simulink model "poco_ref_al_r307"  (Simulink 6.2)
settings: Solver=ode45  StartTime=0.0  StopTime=100000  RelTol=1e-3
libraries: xbsIndex_r3 x1012, xps_library x42, ddc_library x4, adcscope_lib x2, fft_library x2, pfb_library x2, delay_lib x1
(part 7 of 9)

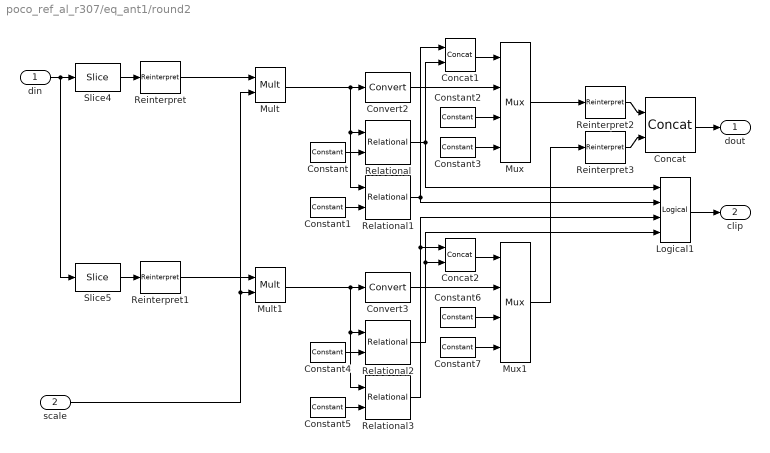
== system poco_ref_al_r307/eq_ant1/round2 ==
  din : Inport  Port=1  LatchInput=off
  scale : Inport  Port=2  LatchInput=off
  Concat : xbsIndex_r3/Concat  num_inputs=2  explicit_period=off  period=1  dbl_ovrd=off
  Concat1 : xbsIndex_r3/Concat  num_inputs=2  explicit_period=off  period=1  dbl_ovrd=off
  Concat2 : xbsIndex_r3/Concat  num_inputs=2  explicit_period=off  period=1  dbl_ovrd=off
  Constant : xbsIndex_r3/Constant  const=7/8  equ=P=C  arith_type="Signed  (2's comp)"  n_bits=27  bin_pt=18  opselect=C  inp2=PCIN>>17  opr=+  inp1=P  carry=CIN  iostate=0  explicit_period=on  period=1  dbl_ovrd=off
  Constant1 : xbsIndex_r3/Constant  const=-7/8  equ=P=C  arith_type="Signed  (2's comp)"  n_bits=27  bin_pt=18  opselect=C  inp2=PCIN>>17  opr=+  inp1=P  carry=CIN  iostate=0  explicit_period=on  period=1  dbl_ovrd=off
  Constant2 : xbsIndex_r3/Constant  const=7/8  equ=P=C  arith_type="Signed  (2's comp)"  n_bits=4  bin_pt=3  opselect=C  inp2=PCIN>>17  opr=+  inp1=P  carry=CIN  iostate=0  explicit_period=on  period=1  dbl_ovrd=off
  Constant3 : xbsIndex_r3/Constant  const=-7/8  equ=P=C  arith_type="Signed  (2's comp)"  n_bits=4  bin_pt=3  opselect=C  inp2=PCIN>>17  opr=+  inp1=P  carry=CIN  iostate=0  explicit_period=on  period=1  dbl_ovrd=off
  Constant4 : xbsIndex_r3/Constant  const=7/8  equ=P=C  arith_type="Signed  (2's comp)"  n_bits=27  bin_pt=18  opselect=C  inp2=PCIN>>17  opr=+  inp1=P  carry=CIN  iostate=0  explicit_period=on  period=1  dbl_ovrd=off
  Constant5 : xbsIndex_r3/Constant  const=-7/8  equ=P=C  arith_type="Signed  (2's comp)"  n_bits=27  bin_pt=18  opselect=C  inp2=PCIN>>17  opr=+  inp1=P  carry=CIN  iostate=0  explicit_period=on  period=1  dbl_ovrd=off
  Constant6 : xbsIndex_r3/Constant  const=7/8  equ=P=C  arith_type="Signed  (2's comp)"  n_bits=4  bin_pt=3  opselect=C  inp2=PCIN>>17  opr=+  inp1=P  carry=CIN  iostate=0  explicit_period=on  period=1  dbl_ovrd=off
  Constant7 : xbsIndex_r3/Constant  const=-7/8  equ=P=C  arith_type="Signed  (2's comp)"  n_bits=4  bin_pt=3  opselect=C  inp2=PCIN>>17  opr=+  inp1=P  carry=CIN  iostate=0  explicit_period=on  period=1  dbl_ovrd=off
  Convert2 : xbsIndex_r3/Convert  arith_type="Signed  (2's comp)"  n_bits=4  bin_pt=3  quantization="Round  (unbiased: Even Values)"  overflow=Wrap  latency=2  explicit_period=off  period=1  dbl_ovrd=off  show_param=off  inserted_by_tool=off  pipeline=off
      settings: xl_area=[0, 0, 0, 0, 0, 0, 0]
  Convert3 : xbsIndex_r3/Convert  arith_type="Signed  (2's comp)"  n_bits=4  bin_pt=3  quantization="Round  (unbiased: Even Values)"  overflow=Wrap  latency=2  explicit_period=off  period=1  dbl_ovrd=off  show_param=off  inserted_by_tool=off  pipeline=off
      settings: xl_area=[0, 0, 0, 0, 0, 0, 0]
  Logical1 : xbsIndex_r3/Logical  logical_function=OR  inputs=4  precision=Full  arith_type=Unsigned  n_bits=8  bin_pt=2  align_bp=on  latency=2  explicit_period=off  period=1  en=off  dbl_ovrd=off  show_param=off
      settings: xl_area=[0, 0, 0, 0, 0, 0, 0]
  Mult : xbsIndex_r3/Mult  precision=Full  arith_type="Signed  (2's comp)"  n_bits=8  bin_pt=2  quantization=Truncate  overflow=Wrap  latency=2  explicit_period=off  period=1  en=off  dbl_ovrd=off  show_param=on  mult_type=Parallel  oversample=2  use_embedded=on  pipeline=on  use_rpm=on  placement_style=Rectangular Shape  gen_core=off
      settings: xl_area=[0, 0, 0, 0, 0, 0, 0]
  Mult1 : xbsIndex_r3/Mult  precision=Full  arith_type="Signed  (2's comp)"  n_bits=8  bin_pt=2  quantization=Truncate  overflow=Wrap  latency=2  explicit_period=off  period=1  en=off  dbl_ovrd=off  show_param=on  mult_type=Parallel  oversample=2  use_embedded=on  pipeline=on  use_rpm=on  placement_style=Rectangular Shape  gen_core=off
      settings: xl_area=[0, 0, 0, 0, 0, 0, 0]
  Mux : xbsIndex_r3/Mux  inputs=3  precision=Full  arith_type="Signed  (2's comp)"  n_bits=8  bin_pt=2  quantization=Truncate  overflow=Wrap  latency=0  explicit_period=off  period=1  en=off  dbl_ovrd=off  show_param=off  mux_type=off  use_rpm=off  gen_core=off
      settings: xl_area=[0, 0, 0, 0, 0, 0, 0]
  Mux1 : xbsIndex_r3/Mux  inputs=3  precision=Full  arith_type="Signed  (2's comp)"  n_bits=8  bin_pt=2  quantization=Truncate  overflow=Wrap  latency=0  explicit_period=off  period=1  en=off  dbl_ovrd=off  show_param=off  mux_type=off  use_rpm=off  gen_core=off
      settings: xl_area=[0, 0, 0, 0, 0, 0, 0]
  Reinterpret : xbsIndex_r3/Reinterpret  force_arith_type=on  arith_type="Signed  (2's comp)"  force_bin_pt=on  bin_pt=17  force_valid=on
  Reinterpret1 : xbsIndex_r3/Reinterpret  force_arith_type=on  arith_type="Signed  (2's comp)"  force_bin_pt=on  bin_pt=17  force_valid=on
  Reinterpret2 : xbsIndex_r3/Reinterpret  force_arith_type=on  arith_type=Unsigned  force_bin_pt=on  bin_pt=0  force_valid=on
  Reinterpret3 : xbsIndex_r3/Reinterpret  force_arith_type=on  arith_type=Unsigned  force_bin_pt=on  bin_pt=0  force_valid=on
  Relational : xbsIndex_r3/Relational  mode=a>b  latency=2  explicit_period=off  period=1  en=off  dbl_ovrd=off  show_param=off
      settings: xl_area=[0, 0, 0, 0, 0, 0, 0]
  Relational1 : xbsIndex_r3/Relational  mode=a<b  latency=2  explicit_period=off  period=1  en=off  dbl_ovrd=off  show_param=off
      settings: xl_area=[0, 0, 0, 0, 0, 0, 0]
  Relational2 : xbsIndex_r3/Relational  mode=a>b  latency=2  explicit_period=off  period=1  en=off  dbl_ovrd=off  show_param=off
      settings: xl_area=[0, 0, 0, 0, 0, 0, 0]
  Relational3 : xbsIndex_r3/Relational  mode=a<b  latency=2  explicit_period=off  period=1  en=off  dbl_ovrd=off  show_param=off
      settings: xl_area=[0, 0, 0, 0, 0, 0, 0]
  Slice4 : xbsIndex_r3/Slice  mode=Upper Bit Location + Width  nbits=18  bit1=0  base1=MSB of Input  bit0=0  base0=LSB of Input  boolean_output=off  explicit_period=off  period=1  dbl_ovrd=off
  Slice5 : xbsIndex_r3/Slice  mode=Lower Bit Location + Width  nbits=18  bit1=0  base1=MSB of Input  bit0=0  base0=LSB of Input  boolean_output=off  explicit_period=off  period=1  dbl_ovrd=off
  dout : Outport
  clip : Outport  Port=2
  wires:
  Logical1/1 -> clip/1
  Mult/1 -> Relational1/1, Relational/1, Convert2/1
  Mult1/1 -> Relational3/1, Relational2/1, Convert3/1
  Mux1/1 -> Reinterpret3/1
  Mux/1 -> Reinterpret2/1
  Relational3/1 -> Logical1/3, Concat2/1
  Relational2/1 -> Logical1/4, Concat2/2
  Constant7/1 -> Mux1/4
  Constant6/1 -> Mux1/3
  Constant5/1 -> Relational3/2
  Constant4/1 -> Relational2/2
  Concat2/1 -> Mux1/1
  Convert3/1 -> Mux1/2
  Relational1/1 -> Logical1/2, Concat1/1
  Relational/1 -> Logical1/1, Concat1/2
  Constant3/1 -> Mux/4
  Constant2/1 -> Mux/3
  Constant1/1 -> Relational1/2
  Constant/1 -> Relational/2
  Concat1/1 -> Mux/1
  Convert2/1 -> Mux/2
  scale/1 -> Mult/2, Mult1/2
  Reinterpret/1 -> Mult/1
  Reinterpret1/1 -> Mult1/1
  Concat/1 -> dout/1
  din/1 -> Slice5/1, Slice4/1
  Reinterpret3/1 -> Concat/2
  Slice5/1 -> Reinterpret1/1
  Reinterpret2/1 -> Concat/1
  Slice4/1 -> Reinterpret/1

== system poco_ref_al_r307/pulse_ext1/posedge ==
  In : Inport  Port=1  LatchInput=off
  Delay : xbsIndex_r3/Delay  latency=1  reg_retiming=off  explicit_period=off  period=1  en=off  accept_only_valid=off  init_zero=on  dbl_ovrd=off  show_param=off
      settings: xl_area=[0, 0, 0, 0, 0, 0, 0]
  Inverter : xbsIndex_r3/Inverter  latency=0  explicit_period=off  period=1  en=off  dbl_ovrd=off  show_param=off
      settings: xl_area=[0, 0, 0, 0, 0, 0, 0]
  Logical : xbsIndex_r3/Logical  logical_function=AND  inputs=2  precision=Full  arith_type=Unsigned  n_bits=8  bin_pt=2  align_bp=on  latency=0  explicit_period=off  period=1  en=off  dbl_ovrd=off  show_param=off
      settings: xl_area=[0, 0, 0, 0, 0, 0, 0]
  Out : Outport
  wires:
  Logical/1 -> Out/1
  In/1 -> Logical/2, Delay/1
  Inverter/1 -> Logical/1
  Delay/1 -> Inverter/1

== system poco_ref_al_r307/pulse_ext2/posedge ==
  In : Inport  Port=1  LatchInput=off
  Delay : xbsIndex_r3/Delay  latency=1  reg_retiming=off  explicit_period=off  period=1  en=off  accept_only_valid=off  init_zero=on  dbl_ovrd=off  show_param=off
      settings: xl_area=[0, 0, 0, 0, 0, 0, 0]
  Inverter : xbsIndex_r3/Inverter  latency=0  explicit_period=off  period=1  en=off  dbl_ovrd=off  show_param=off
      settings: xl_area=[0, 0, 0, 0, 0, 0, 0]
  Logical : xbsIndex_r3/Logical  logical_function=AND  inputs=2  precision=Full  arith_type=Unsigned  n_bits=8  bin_pt=2  align_bp=on  latency=0  explicit_period=off  period=1  en=off  dbl_ovrd=off  show_param=off
      settings: xl_area=[0, 0, 0, 0, 0, 0, 0]
  Out : Outport
  wires:
  Delay/1 -> Inverter/1
  Inverter/1 -> Logical/1
  In/1 -> Delay/1, Logical/2
  Logical/1 -> Out/1

== system poco_ref_al_r307/pulse_ext3/posedge ==
  In : Inport  Port=1  LatchInput=off
  Delay : xbsIndex_r3/Delay  latency=1  reg_retiming=off  explicit_period=off  period=1  en=off  accept_only_valid=off  init_zero=on  dbl_ovrd=off  show_param=off
      settings: xl_area=[0, 0, 0, 0, 0, 0, 0]
  Inverter : xbsIndex_r3/Inverter  latency=0  explicit_period=off  period=1  en=off  dbl_ovrd=off  show_param=off
      settings: xl_area=[0, 0, 0, 0, 0, 0, 0]
  Logical : xbsIndex_r3/Logical  logical_function=AND  inputs=2  precision=Full  arith_type=Unsigned  n_bits=8  bin_pt=2  align_bp=on  latency=0  explicit_period=off  period=1  en=off  dbl_ovrd=off  show_param=off
      settings: xl_area=[0, 0, 0, 0, 0, 0, 0]
  Out : Outport
  wires:
  Delay/1 -> Inverter/1
  Inverter/1 -> Logical/1
  In/1 -> Delay/1, Logical/2
  Logical/1 -> Out/1

== system poco_ref_al_r307/pulse_ext4/posedge ==
  In : Inport  Port=1  LatchInput=off
  Delay : xbsIndex_r3/Delay  latency=1  reg_retiming=off  explicit_period=off  period=1  en=off  accept_only_valid=off  init_zero=on  dbl_ovrd=off  show_param=off
      settings: xl_area=[0, 0, 0, 0, 0, 0, 0]
  Inverter : xbsIndex_r3/Inverter  latency=0  explicit_period=off  period=1  en=off  dbl_ovrd=off  show_param=off
      settings: xl_area=[0, 0, 0, 0, 0, 0, 0]
  Logical : xbsIndex_r3/Logical  logical_function=AND  inputs=2  precision=Full  arith_type=Unsigned  n_bits=8  bin_pt=2  align_bp=on  latency=0  explicit_period=off  period=1  en=off  dbl_ovrd=off  show_param=off
      settings: xl_area=[0, 0, 0, 0, 0, 0, 0]
  Out : Outport
  wires:
  Delay/1 -> Inverter/1
  Inverter/1 -> Logical/1
  In/1 -> Delay/1, Logical/2
  Logical/1 -> Out/1

== system poco_ref_al_r307/pulse_ext5/posedge ==
  In : Inport  Port=1  LatchInput=off
  Delay : xbsIndex_r3/Delay  latency=1  reg_retiming=off  explicit_period=off  period=1  en=off  accept_only_valid=off  init_zero=on  dbl_ovrd=off  show_param=off
      settings: xl_area=[0, 0, 0, 0, 0, 0, 0]
  Inverter : xbsIndex_r3/Inverter  latency=0  explicit_period=off  period=1  en=off  dbl_ovrd=off  show_param=off
      settings: xl_area=[0, 0, 0, 0, 0, 0, 0]
  Logical : xbsIndex_r3/Logical  logical_function=AND  inputs=2  precision=Full  arith_type=Unsigned  n_bits=8  bin_pt=2  align_bp=on  latency=0  explicit_period=off  period=1  en=off  dbl_ovrd=off  show_param=off
      settings: xl_area=[0, 0, 0, 0, 0, 0, 0]
  Out : Outport
  wires:
  Logical/1 -> Out/1
  In/1 -> Logical/2, Delay/1
  Inverter/1 -> Logical/1
  Delay/1 -> Inverter/1

== system poco_ref_al_r307/pulse_ext6/posedge ==
  In : Inport  Port=1  LatchInput=off
  Delay : xbsIndex_r3/Delay  latency=1  reg_retiming=off  explicit_period=off  period=1  en=off  accept_only_valid=off  init_zero=on  dbl_ovrd=off  show_param=off
      settings: xl_area=[0, 0, 0, 0, 0, 0, 0]
  Inverter : xbsIndex_r3/Inverter  latency=0  explicit_period=off  period=1  en=off  dbl_ovrd=off  show_param=off
      settings: xl_area=[0, 0, 0, 0, 0, 0, 0]
  Logical : xbsIndex_r3/Logical  logical_function=AND  inputs=2  precision=Full  arith_type=Unsigned  n_bits=8  bin_pt=2  align_bp=on  latency=0  explicit_period=off  period=1  en=off  dbl_ovrd=off  show_param=off
      settings: xl_area=[0, 0, 0, 0, 0, 0, 0]
  Out : Outport
  wires:
  Logical/1 -> Out/1
  In/1 -> Logical/2, Delay/1
  Inverter/1 -> Logical/1
  Delay/1 -> Inverter/1

== system poco_ref_al_r307/pulse_ext7/posedge ==
  In : Inport  Port=1  LatchInput=off
  Delay : xbsIndex_r3/Delay  latency=1  reg_retiming=off  explicit_period=off  period=1  en=off  accept_only_valid=off  init_zero=on  dbl_ovrd=off  show_param=off
      settings: xl_area=[0, 0, 0, 0, 0, 0, 0]
  Inverter : xbsIndex_r3/Inverter  latency=0  explicit_period=off  period=1  en=off  dbl_ovrd=off  show_param=off
      settings: xl_area=[0, 0, 0, 0, 0, 0, 0]
  Logical : xbsIndex_r3/Logical  logical_function=AND  inputs=2  precision=Full  arith_type=Unsigned  n_bits=8  bin_pt=2  align_bp=on  latency=0  explicit_period=off  period=1  en=off  dbl_ovrd=off  show_param=off
      settings: xl_area=[0, 0, 0, 0, 0, 0, 0]
  Out : Outport
  wires:
  Logical/1 -> Out/1
  In/1 -> Logical/2, Delay/1
  Inverter/1 -> Logical/1
  Delay/1 -> Inverter/1

== system poco_ref_al_r307/sync_gen/edge ==
  in : Inport  Port=1  LatchInput=off
  Delay4 : xbsIndex_r3/Delay  latency=1  reg_retiming=off  explicit_period=off  period=1  en=off  accept_only_valid=off  init_zero=on  dbl_ovrd=off  show_param=off
      settings: xl_area=[0, 0, 0, 0, 0, 0, 0]
  Logical3 : xbsIndex_r3/Logical  logical_function=XOR  inputs=2  precision=Full  arith_type=Unsigned  n_bits=8  bin_pt=2  align_bp=on  latency=0  explicit_period=off  period=1  en=off  dbl_ovrd=off  show_param=off
      settings: xl_area=[0, 0, 0, 0, 0, 0, 0]
  out : Outport
  wires:
  Logical3/1 -> out/1
  Delay4/1 -> Logical3/1
  in/1 -> Delay4/1, Logical3/2

== system poco_ref_al_r307/sync_gen/posedge1 ==
  In : Inport  Port=1  LatchInput=off
  Delay : xbsIndex_r3/Delay  latency=1  reg_retiming=off  explicit_period=off  period=1  en=off  accept_only_valid=off  init_zero=on  dbl_ovrd=off  show_param=off
      settings: xl_area=[0, 0, 0, 0, 0, 0, 0]
  Inverter : xbsIndex_r3/Inverter  latency=0  explicit_period=off  period=1  en=off  dbl_ovrd=off  show_param=off
      settings: xl_area=[0, 0, 0, 0, 0, 0, 0]
  Logical : xbsIndex_r3/Logical  logical_function=AND  inputs=2  precision=Full  arith_type=Unsigned  n_bits=8  bin_pt=2  align_bp=on  latency=0  explicit_period=off  period=1  en=off  dbl_ovrd=off  show_param=off
      settings: xl_area=[0, 0, 0, 0, 0, 0, 0]
  Out : Outport
  wires:
  Logical/1 -> Out/1
  In/1 -> Logical/2, Delay/1
  Inverter/1 -> Logical/1
  Delay/1 -> Inverter/1

== system poco_ref_al_r307/sync_gen/posedge2 ==
  In : Inport  Port=1  LatchInput=off
  Delay : xbsIndex_r3/Delay  latency=1  reg_retiming=off  explicit_period=off  period=1  en=off  accept_only_valid=off  init_zero=on  dbl_ovrd=off  show_param=off
      settings: xl_area=[0, 0, 0, 0, 0, 0, 0]
  Inverter : xbsIndex_r3/Inverter  latency=0  explicit_period=off  period=1  en=off  dbl_ovrd=off  show_param=off
      settings: xl_area=[0, 0, 0, 0, 0, 0, 0]
  Logical : xbsIndex_r3/Logical  logical_function=AND  inputs=2  precision=Full  arith_type=Unsigned  n_bits=8  bin_pt=2  align_bp=on  latency=0  explicit_period=off  period=1  en=off  dbl_ovrd=off  show_param=off
      settings: xl_area=[0, 0, 0, 0, 0, 0, 0]
  Out : Outport
  wires:
  Delay/1 -> Inverter/1
  Inverter/1 -> Logical/1
  In/1 -> Delay/1, Logical/2
  Logical/1 -> Out/1

== system poco_ref_al_r307/dir_x/aa/c_to_ri ==
  c : Inport  Port=1  LatchInput=off
  force_im : xbsIndex_r3/Reinterpret  force_arith_type=on  arith_type="Signed  (2's comp)"  force_bin_pt=on  bin_pt=bin_pt  force_valid=on
  force_re : xbsIndex_r3/Reinterpret  force_arith_type=on  arith_type="Signed  (2's comp)"  force_bin_pt=on  bin_pt=bin_pt  force_valid=on
  slice_im : xbsIndex_r3/Slice  mode=Lower Bit Location + Width  nbits=n_bits  bit1=0  base1=MSB of Input  bit0=0  base0=LSB of Input  boolean_output=off  explicit_period=off  period=1  dbl_ovrd=off
  slice_re : xbsIndex_r3/Slice  mode=Upper Bit Location + Width  nbits=n_bits  bit1=0  base1=MSB of Input  bit0=0  base0=LSB of Input  boolean_output=off  explicit_period=off  period=1  dbl_ovrd=off
  re : Outport
  im : Outport  Port=2
  wires:
  slice_re/1 -> force_re/1
  slice_im/1 -> force_im/1
  force_re/1 -> re/1
  force_im/1 -> im/1
  c/1 -> slice_re/1, slice_im/1

== system poco_ref_al_r307/dir_x/aa/c_to_ri1 ==
  c : Inport  Port=1  LatchInput=off
  force_im : xbsIndex_r3/Reinterpret  force_arith_type=on  arith_type="Signed  (2's comp)"  force_bin_pt=on  bin_pt=bin_pt  force_valid=on
  force_re : xbsIndex_r3/Reinterpret  force_arith_type=on  arith_type="Signed  (2's comp)"  force_bin_pt=on  bin_pt=bin_pt  force_valid=on
  slice_im : xbsIndex_r3/Slice  mode=Lower Bit Location + Width  nbits=n_bits  bit1=0  base1=MSB of Input  bit0=0  base0=LSB of Input  boolean_output=off  explicit_period=off  period=1  dbl_ovrd=off
  slice_re : xbsIndex_r3/Slice  mode=Upper Bit Location + Width  nbits=n_bits  bit1=0  base1=MSB of Input  bit0=0  base0=LSB of Input  boolean_output=off  explicit_period=off  period=1  dbl_ovrd=off
  re : Outport
  im : Outport  Port=2
  wires:
  slice_re/1 -> force_re/1
  slice_im/1 -> force_im/1
  force_re/1 -> re/1
  force_im/1 -> im/1
  c/1 -> slice_re/1, slice_im/1

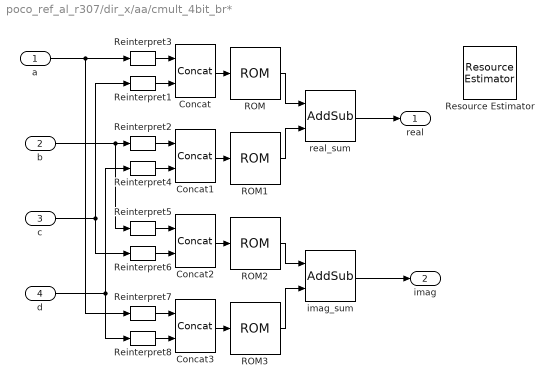
== system poco_ref_al_r307/dir_x/aa/cmult_4bit_br* ==
  a : Inport  Port=1  LatchInput=off
  b : Inport  Port=2  LatchInput=off
  c : Inport  Port=3  LatchInput=off
  d : Inport  Port=4  LatchInput=off
  Concat{,1..3} (4 alike) : xbsIndex_r3/Concat  num_inputs=2  explicit_period=off  period=1  dbl_ovrd=off
  ROM : xbsIndex_r3/ROM  depth=256  initVector=transpose(transpose([0:7 -8:-1]) * [0:7 -8:-1]) / 64  arith_type="Signed  (2's comp)"  n_bits=8  bin_pt=6  latency=mult_latency  init_zero=on  explicit_period=off  period=1  rst=off  init_reg=0  en=off  dbl_ovrd=off  show_param=off  distributed_mem=off  use_rpm=off  gen_core=off
      settings: xl_area=[0 0 1 0 0 0 0]
  ROM1 : xbsIndex_r3/ROM  depth=256  initVector=transpose([0:7 -8:-1]) * [0:7 -8:-1] / 64  arith_type="Signed  (2's comp)"  n_bits=8  bin_pt=6  latency=mult_latency  init_zero=on  explicit_period=off  period=1  rst=off  init_reg=0  en=off  dbl_ovrd=off  show_param=off  distributed_mem=off  use_rpm=off  gen_core=off
      settings: xl_area=[0 0 1 0 0 0 0]
  ROM2 : xbsIndex_r3/ROM  depth=256  initVector=transpose([0:7 -8:-1]) * [0:7 -8:-1] / 64  arith_type="Signed  (2's comp)"  n_bits=8  bin_pt=6  latency=mult_latency  init_zero=on  explicit_period=off  period=1  rst=off  init_reg=0  en=off  dbl_ovrd=off  show_param=off  distributed_mem=off  use_rpm=off  gen_core=off
      settings: xl_area=[0 0 1 0 0 0 0]
  ROM3 : xbsIndex_r3/ROM  depth=256  initVector=transpose([0:7 -8:-1]) * [0:7 -8:-1] / 64  arith_type="Signed  (2's comp)"  n_bits=8  bin_pt=6  latency=mult_latency  init_zero=on  explicit_period=off  period=1  rst=off  init_reg=0  en=off  dbl_ovrd=off  show_param=off  distributed_mem=off  use_rpm=off  gen_core=off
      settings: xl_area=[0 0 1 0 0 0 0]
  Reinterpret{1..8} (8 alike) : xbsIndex_r3/Reinterpret  force_arith_type=on  arith_type=Unsigned  force_bin_pt=on  bin_pt=0  force_valid=on
  Resource Estimator : xbsIndex_r3/Resource Estimator  Tag=resEstTag  xl_estimator_area=[10 18 4 16 0 0 0]  xl_use_estimator_area=off  simulink_period=1  mrp_directory=B:\projects\eor_eight_station
      settings: AttributesFormatString=Resource\nEstimator
  imag_sum : xbsIndex_r3/AddSub  mode=Subtraction  precision=Full  arith_type=Unsigned  n_bits=8  bin_pt=2  quantization=Truncate  overflow=Wrap  latency=add_latency  explicit_period=off  period=1  use_carryin=off  use_carryout=off  en=off  dbl_ovrd=off  show_param=off  use_core=on  pipeline=off  use_rpm=on  gen_core=off
      settings: xl_area=[5 9 0 8 0 0 0]
  real_sum : xbsIndex_r3/AddSub  mode=Addition  precision=Full  arith_type=Unsigned  n_bits=8  bin_pt=2  quantization=Truncate  overflow=Wrap  latency=add_latency  explicit_period=off  period=1  use_carryin=off  use_carryout=off  en=off  dbl_ovrd=off  show_param=off  use_core=on  pipeline=off  use_rpm=on  gen_core=off
      settings: xl_area=[5 9 0 8 0 0 0]
  real : Outport
  imag : Outport  Port=2
  wires:
  Reinterpret8/1 -> Concat3/2
  Reinterpret7/1 -> Concat3/1
  Reinterpret6/1 -> Concat2/2
  Reinterpret5/1 -> Concat2/1
  Reinterpret4/1 -> Concat1/2
  Reinterpret2/1 -> Concat1/1
  Reinterpret1/1 -> Concat/2
  Reinterpret3/1 -> Concat/1
  Concat3/1 -> ROM3/1
  Concat2/1 -> ROM2/1
  Concat1/1 -> ROM1/1
  Concat/1 -> ROM/1
  imag_sum/1 -> imag/1
  real_sum/1 -> real/1
  d/1 -> Reinterpret8/1, Reinterpret4/1
  b/1 -> Reinterpret5/1, Reinterpret2/1
  c/1 -> Reinterpret6/1, Reinterpret1/1
  a/1 -> Reinterpret7/1, Reinterpret3/1
  ROM3/1 -> imag_sum/2
  ROM2/1 -> imag_sum/1
  ROM1/1 -> real_sum/2
  ROM/1 -> real_sum/1

== system poco_ref_al_r307/dir_x/aa/vacc_32bit ==
  din : Inport  Port=1  LatchInput=off
  new_acc : Inport  Port=2  LatchInput=off
  Adder0 : xbsIndex_r3/AddSub  mode=Addition  precision=User Defined  arith_type="Signed  (2's comp)"  n_bits=32  bin_pt=6  quantization=Truncate  overflow=Wrap  latency=2  explicit_period=on  period=1  use_carryin=off  use_carryout=off  en=off  dbl_ovrd=off  show_param=off  use_core=on  pipeline=off  use_rpm=on  gen_core=off
      settings: xl_area=[0, 0, 0, 0, 0, 0, 0]
  Mux0 : xbsIndex_r3/Mux  inputs=2  precision=Full  arith_type="Signed  (2's comp)"  n_bits=8  bin_pt=2  quantization=Truncate  overflow=Wrap  latency=0  explicit_period=off  period=1  en=off  dbl_ovrd=off  show_param=off  mux_type=off  use_rpm=off  gen_core=off
      settings: xl_area=[0, 0, 0, 0, 0, 0, 0]
  delay_bram : Subsystem  mask(delay_bram){DelayLen=n_chans - 2, bram_latency=2}
      mask prompts: DelayLen "Delay By:"; bram_latency "BRAM Latency"
      mask help: A delay block that uses BRAM for its storage.
      mask init:
      | if (DelayLen <= bram_latency)
      | 	error('delay value must be greater than BRAM Latency');
      | end
      | BitWidth = max(ceil(log2(DelayLen)), 2);
      mask Help: eval('xlWeb([getenv(''MLIB_ROOT''), ''\doc\html\sp_delay_bram\sp_delay_bram.html''])')
  pulse_ext : Subsystem  mask(pulse_ext){pulse_len=n_chans}
      mask prompts: pulse_len "Length of Pulse"
      mask help:
      | Extends a boolean signal to be high for the specified number of clocks after
      | the last high input.
      mask init:
      | bits = ceil(log2(pulse_len+1));
      mask Help: eval('xlWeb([getenv(''MLIB_ROOT''), ''\casper_library\doc\pulse_ext_usage.html''])')
  zero : xbsIndex_r3/Constant  const=0  equ=P=C  arith_type="Signed  (2's comp)"  n_bits=32  bin_pt=6  opselect=C  inp2=PCIN>>17  opr=+  inp1=P  carry=CIN  iostate=0  explicit_period=on  period=1  dbl_ovrd=off
  dout : Outport
  valid : Outport  Port=2
  wires:
  Adder0/1 -> delay_bram/1(In1)
  delay_bram/1(Out1) -> dout/1, Mux0/2
  new_acc/1 -> pulse_ext/1(in)
  din/1 -> Adder0/1
  pulse_ext/1(out) -> valid/1, Mux0/1
  Mux0/1 -> Adder0/2
  zero/1 -> Mux0/3

== system poco_ref_al_r307/dir_x/ab/c_to_ri ==
  c : Inport  Port=1  LatchInput=off
  force_im : xbsIndex_r3/Reinterpret  force_arith_type=on  arith_type="Signed  (2's comp)"  force_bin_pt=on  bin_pt=bin_pt  force_valid=on
  force_re : xbsIndex_r3/Reinterpret  force_arith_type=on  arith_type="Signed  (2's comp)"  force_bin_pt=on  bin_pt=bin_pt  force_valid=on
  slice_im : xbsIndex_r3/Slice  mode=Lower Bit Location + Width  nbits=n_bits  bit1=0  base1=MSB of Input  bit0=0  base0=LSB of Input  boolean_output=off  explicit_period=off  period=1  dbl_ovrd=off
  slice_re : xbsIndex_r3/Slice  mode=Upper Bit Location + Width  nbits=n_bits  bit1=0  base1=MSB of Input  bit0=0  base0=LSB of Input  boolean_output=off  explicit_period=off  period=1  dbl_ovrd=off
  re : Outport
  im : Outport  Port=2
  wires:
  c/1 -> slice_im/1, slice_re/1
  force_im/1 -> im/1
  force_re/1 -> re/1
  slice_im/1 -> force_im/1
  slice_re/1 -> force_re/1

== system poco_ref_al_r307/dir_x/ab/c_to_ri1 ==
  c : Inport  Port=1  LatchInput=off
  force_im : xbsIndex_r3/Reinterpret  force_arith_type=on  arith_type="Signed  (2's comp)"  force_bin_pt=on  bin_pt=bin_pt  force_valid=on
  force_re : xbsIndex_r3/Reinterpret  force_arith_type=on  arith_type="Signed  (2's comp)"  force_bin_pt=on  bin_pt=bin_pt  force_valid=on
  slice_im : xbsIndex_r3/Slice  mode=Lower Bit Location + Width  nbits=n_bits  bit1=0  base1=MSB of Input  bit0=0  base0=LSB of Input  boolean_output=off  explicit_period=off  period=1  dbl_ovrd=off
  slice_re : xbsIndex_r3/Slice  mode=Upper Bit Location + Width  nbits=n_bits  bit1=0  base1=MSB of Input  bit0=0  base0=LSB of Input  boolean_output=off  explicit_period=off  period=1  dbl_ovrd=off
  re : Outport
  im : Outport  Port=2
  wires:
  c/1 -> slice_im/1, slice_re/1
  force_im/1 -> im/1
  force_re/1 -> re/1
  slice_im/1 -> force_im/1
  slice_re/1 -> force_re/1

== system poco_ref_al_r307/dir_x/ab/cmult_4bit_sl* ==
  a : Inport  Port=1  LatchInput=off
  b : Inport  Port=2  LatchInput=off
  c : Inport  Port=3  LatchInput=off
  d : Inport  Port=4  LatchInput=off
  ac : xbsIndex_r3/Mult  precision=Full  arith_type="Signed  (2's comp)"  n_bits=7  bin_pt=6  quantization=Truncate  overflow=Wrap  latency=mult_latency  explicit_period=off  period=1  en=off  dbl_ovrd=off  show_param=on  mult_type=Parallel  oversample=2  use_embedded=off  pipeline=off  use_rpm=on  placement_style=Rectangular Shape  gen_core=off
      settings: xl_area=[10 7 0 17 0 0 0]
  ad : xbsIndex_r3/Mult  precision=Full  arith_type="Signed  (2's comp)"  n_bits=7  bin_pt=6  quantization=Truncate  overflow=Wrap  latency=mult_latency  explicit_period=off  period=1  en=off  dbl_ovrd=off  show_param=on  mult_type=Parallel  oversample=2  use_embedded=off  pipeline=off  use_rpm=on  placement_style=Rectangular Shape  gen_core=off
      settings: xl_area=[10 7 0 17 0 0 0]
  bc : xbsIndex_r3/Mult  precision=Full  arith_type="Signed  (2's comp)"  n_bits=7  bin_pt=6  quantization=Truncate  overflow=Wrap  latency=mult_latency  explicit_period=off  period=1  en=off  dbl_ovrd=off  show_param=on  mult_type=Parallel  oversample=2  use_embedded=off  pipeline=off  use_rpm=on  placement_style=Rectangular Shape  gen_core=off
      settings: xl_area=[10 7 0 17 0 0 0]
  bd : xbsIndex_r3/Mult  precision=Full  arith_type="Signed  (2's comp)"  n_bits=7  bin_pt=6  quantization=Truncate  overflow=Wrap  latency=mult_latency  explicit_period=off  period=1  en=off  dbl_ovrd=off  show_param=on  mult_type=Parallel  oversample=2  use_embedded=off  pipeline=off  use_rpm=on  placement_style=Rectangular Shape  gen_core=off
      settings: xl_area=[10 7 0 17 0 0 0]
  imag_sum : xbsIndex_r3/AddSub  mode=Subtraction  precision=Full  arith_type=Unsigned  n_bits=8  bin_pt=2  quantization=Truncate  overflow=Wrap  latency=add_latency  explicit_period=off  period=1  use_carryin=off  use_carryout=off  en=off  dbl_ovrd=off  show_param=off  use_core=on  pipeline=off  use_rpm=on  gen_core=off
      settings: xl_area=[4 8 0 7 0 0 0]
  real_sum : xbsIndex_r3/AddSub  mode=Addition  precision=Full  arith_type=Unsigned  n_bits=8  bin_pt=2  quantization=Truncate  overflow=Wrap  latency=add_latency  explicit_period=off  period=1  use_carryin=off  use_carryout=off  en=off  dbl_ovrd=off  show_param=off  use_core=on  pipeline=off  use_rpm=on  gen_core=off
      settings: xl_area=[4 8 0 7 0 0 0]
  real : Outport
  imag : Outport  Port=2
  wires:
  ac/1 -> real_sum/1
  bd/1 -> real_sum/2
  bc/1 -> imag_sum/1
  ad/1 -> imag_sum/2
  a/1 -> ad/1, ac/1
  c/1 -> bc/2, ac/2
  b/1 -> bc/1, bd/1
  d/1 -> ad/2, bd/2
  real_sum/1 -> real/1
  imag_sum/1 -> imag/1

== system poco_ref_al_r307/dir_x/ab/vacc_0 ==
  din : Inport  Port=1  LatchInput=off
  new_acc : Inport  Port=2  LatchInput=off
  Adder0 : xbsIndex_r3/AddSub  mode=Addition  precision=User Defined  arith_type="Signed  (2's comp)"  n_bits=32  bin_pt=6  quantization=Truncate  overflow=Wrap  latency=2  explicit_period=on  period=1  use_carryin=off  use_carryout=off  en=off  dbl_ovrd=off  show_param=off  use_core=on  pipeline=off  use_rpm=on  gen_core=off
      settings: xl_area=[0, 0, 0, 0, 0, 0, 0]
  Mux0 : xbsIndex_r3/Mux  inputs=2  precision=Full  arith_type="Signed  (2's comp)"  n_bits=8  bin_pt=2  quantization=Truncate  overflow=Wrap  latency=0  explicit_period=off  period=1  en=off  dbl_ovrd=off  show_param=off  mux_type=off  use_rpm=off  gen_core=off
      settings: xl_area=[0, 0, 0, 0, 0, 0, 0]
  delay_bram : Subsystem  mask(delay_bram){DelayLen=n_chans - 2, bram_latency=2}
      mask prompts: DelayLen "Delay By:"; bram_latency "BRAM Latency"
      mask help: A delay block that uses BRAM for its storage.
      mask init:
      | if (DelayLen <= bram_latency)
      | 	error('delay value must be greater than BRAM Latency');
      | end
      | BitWidth = max(ceil(log2(DelayLen)), 2);
      mask Help: eval('xlWeb([getenv(''MLIB_ROOT''), ''\doc\html\sp_delay_bram\sp_delay_bram.html''])')
  pulse_ext : Subsystem  mask(pulse_ext){pulse_len=n_chans}
      mask prompts: pulse_len "Length of Pulse"
      mask help:
      | Extends a boolean signal to be high for the specified number of clocks after
      | the last high input.
      mask init:
      | bits = ceil(log2(pulse_len+1));
      mask Help: eval('xlWeb([getenv(''MLIB_ROOT''), ''\casper_library\doc\pulse_ext_usage.html''])')
  zero : xbsIndex_r3/Constant  const=0  equ=P=C  arith_type="Signed  (2's comp)"  n_bits=32  bin_pt=6  opselect=C  inp2=PCIN>>17  opr=+  inp1=P  carry=CIN  iostate=0  explicit_period=on  period=1  dbl_ovrd=off
  dout : Outport
  valid : Outport  Port=2
  wires:
  zero/1 -> Mux0/3
  Mux0/1 -> Adder0/2
  pulse_ext/1(out) -> Mux0/1, valid/1
  din/1 -> Adder0/1
  new_acc/1 -> pulse_ext/1(in)
  Adder0/1 -> delay_bram/1(In1)
  delay_bram/1(Out1) -> dout/1, Mux0/2

== system poco_ref_al_r307/dir_x/ab/vacc_1 ==
  din : Inport  Port=1  LatchInput=off
  new_acc : Inport  Port=2  LatchInput=off
  Adder0 : xbsIndex_r3/AddSub  mode=Addition  precision=User Defined  arith_type="Signed  (2's comp)"  n_bits=32  bin_pt=6  quantization=Truncate  overflow=Wrap  latency=2  explicit_period=on  period=1  use_carryin=off  use_carryout=off  en=off  dbl_ovrd=off  show_param=off  use_core=on  pipeline=off  use_rpm=on  gen_core=off
      settings: xl_area=[0, 0, 0, 0, 0, 0, 0]
  Mux0 : xbsIndex_r3/Mux  inputs=2  precision=Full  arith_type="Signed  (2's comp)"  n_bits=8  bin_pt=2  quantization=Truncate  overflow=Wrap  latency=0  explicit_period=off  period=1  en=off  dbl_ovrd=off  show_param=off  mux_type=off  use_rpm=off  gen_core=off
      settings: xl_area=[0, 0, 0, 0, 0, 0, 0]
  delay_bram : Subsystem  mask(delay_bram){DelayLen=n_chans - 2, bram_latency=2}
      mask prompts: DelayLen "Delay By:"; bram_latency "BRAM Latency"
      mask help: A delay block that uses BRAM for its storage.
      mask init:
      | if (DelayLen <= bram_latency)
      | 	error('delay value must be greater than BRAM Latency');
      | end
      | BitWidth = max(ceil(log2(DelayLen)), 2);
      mask Help: eval('xlWeb([getenv(''MLIB_ROOT''), ''\doc\html\sp_delay_bram\sp_delay_bram.html''])')
  pulse_ext : Subsystem  mask(pulse_ext){pulse_len=n_chans}
      mask prompts: pulse_len "Length of Pulse"
      mask help:
      | Extends a boolean signal to be high for the specified number of clocks after
      | the last high input.
      mask init:
      | bits = ceil(log2(pulse_len+1));
      mask Help: eval('xlWeb([getenv(''MLIB_ROOT''), ''\casper_library\doc\pulse_ext_usage.html''])')
  zero : xbsIndex_r3/Constant  const=0  equ=P=C  arith_type="Signed  (2's comp)"  n_bits=32  bin_pt=6  opselect=C  inp2=PCIN>>17  opr=+  inp1=P  carry=CIN  iostate=0  explicit_period=on  period=1  dbl_ovrd=off
  dout : Outport
  valid : Outport  Port=2
  wires:
  delay_bram/1(Out1) -> Mux0/2, dout/1
  Adder0/1 -> delay_bram/1(In1)
  new_acc/1 -> pulse_ext/1(in)
  din/1 -> Adder0/1
  pulse_ext/1(out) -> valid/1, Mux0/1
  Mux0/1 -> Adder0/2
  zero/1 -> Mux0/3

== system poco_ref_al_r307/dir_x/ac/c_to_ri ==
  c : Inport  Port=1  LatchInput=off
  force_im : xbsIndex_r3/Reinterpret  force_arith_type=on  arith_type="Signed  (2's comp)"  force_bin_pt=on  bin_pt=bin_pt  force_valid=on
  force_re : xbsIndex_r3/Reinterpret  force_arith_type=on  arith_type="Signed  (2's comp)"  force_bin_pt=on  bin_pt=bin_pt  force_valid=on
  slice_im : xbsIndex_r3/Slice  mode=Lower Bit Location + Width  nbits=n_bits  bit1=0  base1=MSB of Input  bit0=0  base0=LSB of Input  boolean_output=off  explicit_period=off  period=1  dbl_ovrd=off
  slice_re : xbsIndex_r3/Slice  mode=Upper Bit Location + Width  nbits=n_bits  bit1=0  base1=MSB of Input  bit0=0  base0=LSB of Input  boolean_output=off  explicit_period=off  period=1  dbl_ovrd=off
  re : Outport
  im : Outport  Port=2
  wires:
  slice_re/1 -> force_re/1
  slice_im/1 -> force_im/1
  force_re/1 -> re/1
  force_im/1 -> im/1
  c/1 -> slice_re/1, slice_im/1

== system poco_ref_al_r307/dir_x/ac/c_to_ri1 ==
  c : Inport  Port=1  LatchInput=off
  force_im : xbsIndex_r3/Reinterpret  force_arith_type=on  arith_type="Signed  (2's comp)"  force_bin_pt=on  bin_pt=bin_pt  force_valid=on
  force_re : xbsIndex_r3/Reinterpret  force_arith_type=on  arith_type="Signed  (2's comp)"  force_bin_pt=on  bin_pt=bin_pt  force_valid=on
  slice_im : xbsIndex_r3/Slice  mode=Lower Bit Location + Width  nbits=n_bits  bit1=0  base1=MSB of Input  bit0=0  base0=LSB of Input  boolean_output=off  explicit_period=off  period=1  dbl_ovrd=off
  slice_re : xbsIndex_r3/Slice  mode=Upper Bit Location + Width  nbits=n_bits  bit1=0  base1=MSB of Input  bit0=0  base0=LSB of Input  boolean_output=off  explicit_period=off  period=1  dbl_ovrd=off
  re : Outport
  im : Outport  Port=2
  wires:
  slice_re/1 -> force_re/1
  slice_im/1 -> force_im/1
  force_re/1 -> re/1
  force_im/1 -> im/1
  c/1 -> slice_re/1, slice_im/1

== system poco_ref_al_r307/dir_x/ac/cmult_4bit_sl* ==
  a : Inport  Port=1  LatchInput=off
  b : Inport  Port=2  LatchInput=off
  c : Inport  Port=3  LatchInput=off
  d : Inport  Port=4  LatchInput=off
  ac : xbsIndex_r3/Mult  precision=Full  arith_type="Signed  (2's comp)"  n_bits=7  bin_pt=6  quantization=Truncate  overflow=Wrap  latency=mult_latency  explicit_period=off  period=1  en=off  dbl_ovrd=off  show_param=on  mult_type=Parallel  oversample=2  use_embedded=off  pipeline=off  use_rpm=on  placement_style=Rectangular Shape  gen_core=off
      settings: xl_area=[10 7 0 17 0 0 0]
  ad : xbsIndex_r3/Mult  precision=Full  arith_type="Signed  (2's comp)"  n_bits=7  bin_pt=6  quantization=Truncate  overflow=Wrap  latency=mult_latency  explicit_period=off  period=1  en=off  dbl_ovrd=off  show_param=on  mult_type=Parallel  oversample=2  use_embedded=off  pipeline=off  use_rpm=on  placement_style=Rectangular Shape  gen_core=off
      settings: xl_area=[10 7 0 17 0 0 0]
  bc : xbsIndex_r3/Mult  precision=Full  arith_type="Signed  (2's comp)"  n_bits=7  bin_pt=6  quantization=Truncate  overflow=Wrap  latency=mult_latency  explicit_period=off  period=1  en=off  dbl_ovrd=off  show_param=on  mult_type=Parallel  oversample=2  use_embedded=off  pipeline=off  use_rpm=on  placement_style=Rectangular Shape  gen_core=off
      settings: xl_area=[10 7 0 17 0 0 0]
  bd : xbsIndex_r3/Mult  precision=Full  arith_type="Signed  (2's comp)"  n_bits=7  bin_pt=6  quantization=Truncate  overflow=Wrap  latency=mult_latency  explicit_period=off  period=1  en=off  dbl_ovrd=off  show_param=on  mult_type=Parallel  oversample=2  use_embedded=off  pipeline=off  use_rpm=on  placement_style=Rectangular Shape  gen_core=off
      settings: xl_area=[10 7 0 17 0 0 0]
  imag_sum : xbsIndex_r3/AddSub  mode=Subtraction  precision=Full  arith_type=Unsigned  n_bits=8  bin_pt=2  quantization=Truncate  overflow=Wrap  latency=add_latency  explicit_period=off  period=1  use_carryin=off  use_carryout=off  en=off  dbl_ovrd=off  show_param=off  use_core=on  pipeline=off  use_rpm=on  gen_core=off
      settings: xl_area=[4 8 0 7 0 0 0]
  real_sum : xbsIndex_r3/AddSub  mode=Addition  precision=Full  arith_type=Unsigned  n_bits=8  bin_pt=2  quantization=Truncate  overflow=Wrap  latency=add_latency  explicit_period=off  period=1  use_carryin=off  use_carryout=off  en=off  dbl_ovrd=off  show_param=off  use_core=on  pipeline=off  use_rpm=on  gen_core=off
      settings: xl_area=[4 8 0 7 0 0 0]
  real : Outport
  imag : Outport  Port=2
  wires:
  imag_sum/1 -> imag/1
  real_sum/1 -> real/1
  d/1 -> bd/2, ad/2
  b/1 -> bd/1, bc/1
  c/1 -> ac/2, bc/2
  a/1 -> ac/1, ad/1
  ad/1 -> imag_sum/2
  bc/1 -> imag_sum/1
  bd/1 -> real_sum/2
  ac/1 -> real_sum/1

== system poco_ref_al_r307/dir_x/ac/vacc_0 ==
  din : Inport  Port=1  LatchInput=off
  new_acc : Inport  Port=2  LatchInput=off
  Adder0 : xbsIndex_r3/AddSub  mode=Addition  precision=User Defined  arith_type="Signed  (2's comp)"  n_bits=32  bin_pt=6  quantization=Truncate  overflow=Wrap  latency=2  explicit_period=on  period=1  use_carryin=off  use_carryout=off  en=off  dbl_ovrd=off  show_param=off  use_core=on  pipeline=off  use_rpm=on  gen_core=off
      settings: xl_area=[0, 0, 0, 0, 0, 0, 0]
  Mux0 : xbsIndex_r3/Mux  inputs=2  precision=Full  arith_type="Signed  (2's comp)"  n_bits=8  bin_pt=2  quantization=Truncate  overflow=Wrap  latency=0  explicit_period=off  period=1  en=off  dbl_ovrd=off  show_param=off  mux_type=off  use_rpm=off  gen_core=off
      settings: xl_area=[0, 0, 0, 0, 0, 0, 0]
  delay_bram : Subsystem  mask(delay_bram){DelayLen=n_chans - 2, bram_latency=2}
      mask prompts: DelayLen "Delay By:"; bram_latency "BRAM Latency"
      mask help: A delay block that uses BRAM for its storage.
      mask init:
      | if (DelayLen <= bram_latency)
      | 	error('delay value must be greater than BRAM Latency');
      | end
      | BitWidth = max(ceil(log2(DelayLen)), 2);
      mask Help: eval('xlWeb([getenv(''MLIB_ROOT''), ''\doc\html\sp_delay_bram\sp_delay_bram.html''])')
  pulse_ext : Subsystem  mask(pulse_ext){pulse_len=n_chans}
      mask prompts: pulse_len "Length of Pulse"
      mask help:
      | Extends a boolean signal to be high for the specified number of clocks after
      | the last high input.
      mask init:
      | bits = ceil(log2(pulse_len+1));
      mask Help: eval('xlWeb([getenv(''MLIB_ROOT''), ''\casper_library\doc\pulse_ext_usage.html''])')
  zero : xbsIndex_r3/Constant  const=0  equ=P=C  arith_type="Signed  (2's comp)"  n_bits=32  bin_pt=6  opselect=C  inp2=PCIN>>17  opr=+  inp1=P  carry=CIN  iostate=0  explicit_period=on  period=1  dbl_ovrd=off
  dout : Outport
  valid : Outport  Port=2
  wires:
  zero/1 -> Mux0/3
  Mux0/1 -> Adder0/2
  pulse_ext/1(out) -> Mux0/1, valid/1
  din/1 -> Adder0/1
  new_acc/1 -> pulse_ext/1(in)
  Adder0/1 -> delay_bram/1(In1)
  delay_bram/1(Out1) -> dout/1, Mux0/2

== system poco_ref_al_r307/dir_x/ac/vacc_1 ==
  din : Inport  Port=1  LatchInput=off
  new_acc : Inport  Port=2  LatchInput=off
  Adder0 : xbsIndex_r3/AddSub  mode=Addition  precision=User Defined  arith_type="Signed  (2's comp)"  n_bits=32  bin_pt=6  quantization=Truncate  overflow=Wrap  latency=2  explicit_period=on  period=1  use_carryin=off  use_carryout=off  en=off  dbl_ovrd=off  show_param=off  use_core=on  pipeline=off  use_rpm=on  gen_core=off
      settings: xl_area=[0, 0, 0, 0, 0, 0, 0]
  Mux0 : xbsIndex_r3/Mux  inputs=2  precision=Full  arith_type="Signed  (2's comp)"  n_bits=8  bin_pt=2  quantization=Truncate  overflow=Wrap  latency=0  explicit_period=off  period=1  en=off  dbl_ovrd=off  show_param=off  mux_type=off  use_rpm=off  gen_core=off
      settings: xl_area=[0, 0, 0, 0, 0, 0, 0]
  delay_bram : Subsystem  mask(delay_bram){DelayLen=n_chans - 2, bram_latency=2}
      mask prompts: DelayLen "Delay By:"; bram_latency "BRAM Latency"
      mask help: A delay block that uses BRAM for its storage.
      mask init:
      | if (DelayLen <= bram_latency)
      | 	error('delay value must be greater than BRAM Latency');
      | end
      | BitWidth = max(ceil(log2(DelayLen)), 2);
      mask Help: eval('xlWeb([getenv(''MLIB_ROOT''), ''\doc\html\sp_delay_bram\sp_delay_bram.html''])')
  pulse_ext : Subsystem  mask(pulse_ext){pulse_len=n_chans}
      mask prompts: pulse_len "Length of Pulse"
      mask help:
      | Extends a boolean signal to be high for the specified number of clocks after
      | the last high input.
      mask init:
      | bits = ceil(log2(pulse_len+1));
      mask Help: eval('xlWeb([getenv(''MLIB_ROOT''), ''\casper_library\doc\pulse_ext_usage.html''])')
  zero : xbsIndex_r3/Constant  const=0  equ=P=C  arith_type="Signed  (2's comp)"  n_bits=32  bin_pt=6  opselect=C  inp2=PCIN>>17  opr=+  inp1=P  carry=CIN  iostate=0  explicit_period=on  period=1  dbl_ovrd=off
  dout : Outport
  valid : Outport  Port=2
  wires:
  delay_bram/1(Out1) -> Mux0/2, dout/1
  Adder0/1 -> delay_bram/1(In1)
  new_acc/1 -> pulse_ext/1(in)
  din/1 -> Adder0/1
  pulse_ext/1(out) -> valid/1, Mux0/1
  Mux0/1 -> Adder0/2
  zero/1 -> Mux0/3

== system poco_ref_al_r307/dir_x/ad/c_to_ri ==
  c : Inport  Port=1  LatchInput=off
  force_im : xbsIndex_r3/Reinterpret  force_arith_type=on  arith_type="Signed  (2's comp)"  force_bin_pt=on  bin_pt=bin_pt  force_valid=on
  force_re : xbsIndex_r3/Reinterpret  force_arith_type=on  arith_type="Signed  (2's comp)"  force_bin_pt=on  bin_pt=bin_pt  force_valid=on
  slice_im : xbsIndex_r3/Slice  mode=Lower Bit Location + Width  nbits=n_bits  bit1=0  base1=MSB of Input  bit0=0  base0=LSB of Input  boolean_output=off  explicit_period=off  period=1  dbl_ovrd=off
  slice_re : xbsIndex_r3/Slice  mode=Upper Bit Location + Width  nbits=n_bits  bit1=0  base1=MSB of Input  bit0=0  base0=LSB of Input  boolean_output=off  explicit_period=off  period=1  dbl_ovrd=off
  re : Outport
  im : Outport  Port=2
  wires:
  c/1 -> slice_im/1, slice_re/1
  force_im/1 -> im/1
  force_re/1 -> re/1
  slice_im/1 -> force_im/1
  slice_re/1 -> force_re/1

== system poco_ref_al_r307/dir_x/ad/c_to_ri1 ==
  c : Inport  Port=1  LatchInput=off
  force_im : xbsIndex_r3/Reinterpret  force_arith_type=on  arith_type="Signed  (2's comp)"  force_bin_pt=on  bin_pt=bin_pt  force_valid=on
  force_re : xbsIndex_r3/Reinterpret  force_arith_type=on  arith_type="Signed  (2's comp)"  force_bin_pt=on  bin_pt=bin_pt  force_valid=on
  slice_im : xbsIndex_r3/Slice  mode=Lower Bit Location + Width  nbits=n_bits  bit1=0  base1=MSB of Input  bit0=0  base0=LSB of Input  boolean_output=off  explicit_period=off  period=1  dbl_ovrd=off
  slice_re : xbsIndex_r3/Slice  mode=Upper Bit Location + Width  nbits=n_bits  bit1=0  base1=MSB of Input  bit0=0  base0=LSB of Input  boolean_output=off  explicit_period=off  period=1  dbl_ovrd=off
  re : Outport
  im : Outport  Port=2
  wires:
  c/1 -> slice_im/1, slice_re/1
  force_im/1 -> im/1
  force_re/1 -> re/1
  slice_im/1 -> force_im/1
  slice_re/1 -> force_re/1

== system poco_ref_al_r307/dir_x/ad/cmult_4bit_sl* ==
  a : Inport  Port=1  LatchInput=off
  b : Inport  Port=2  LatchInput=off
  c : Inport  Port=3  LatchInput=off
  d : Inport  Port=4  LatchInput=off
  ac : xbsIndex_r3/Mult  precision=Full  arith_type="Signed  (2's comp)"  n_bits=7  bin_pt=6  quantization=Truncate  overflow=Wrap  latency=mult_latency  explicit_period=off  period=1  en=off  dbl_ovrd=off  show_param=on  mult_type=Parallel  oversample=2  use_embedded=off  pipeline=off  use_rpm=on  placement_style=Rectangular Shape  gen_core=off
      settings: xl_area=[10 7 0 17 0 0 0]
  ad : xbsIndex_r3/Mult  precision=Full  arith_type="Signed  (2's comp)"  n_bits=7  bin_pt=6  quantization=Truncate  overflow=Wrap  latency=mult_latency  explicit_period=off  period=1  en=off  dbl_ovrd=off  show_param=on  mult_type=Parallel  oversample=2  use_embedded=off  pipeline=off  use_rpm=on  placement_style=Rectangular Shape  gen_core=off
      settings: xl_area=[10 7 0 17 0 0 0]
  bc : xbsIndex_r3/Mult  precision=Full  arith_type="Signed  (2's comp)"  n_bits=7  bin_pt=6  quantization=Truncate  overflow=Wrap  latency=mult_latency  explicit_period=off  period=1  en=off  dbl_ovrd=off  show_param=on  mult_type=Parallel  oversample=2  use_embedded=off  pipeline=off  use_rpm=on  placement_style=Rectangular Shape  gen_core=off
      settings: xl_area=[10 7 0 17 0 0 0]
  bd : xbsIndex_r3/Mult  precision=Full  arith_type="Signed  (2's comp)"  n_bits=7  bin_pt=6  quantization=Truncate  overflow=Wrap  latency=mult_latency  explicit_period=off  period=1  en=off  dbl_ovrd=off  show_param=on  mult_type=Parallel  oversample=2  use_embedded=off  pipeline=off  use_rpm=on  placement_style=Rectangular Shape  gen_core=off
      settings: xl_area=[10 7 0 17 0 0 0]
  imag_sum : xbsIndex_r3/AddSub  mode=Subtraction  precision=Full  arith_type=Unsigned  n_bits=8  bin_pt=2  quantization=Truncate  overflow=Wrap  latency=add_latency  explicit_period=off  period=1  use_carryin=off  use_carryout=off  en=off  dbl_ovrd=off  show_param=off  use_core=on  pipeline=off  use_rpm=on  gen_core=off
      settings: xl_area=[4 8 0 7 0 0 0]
  real_sum : xbsIndex_r3/AddSub  mode=Addition  precision=Full  arith_type=Unsigned  n_bits=8  bin_pt=2  quantization=Truncate  overflow=Wrap  latency=add_latency  explicit_period=off  period=1  use_carryin=off  use_carryout=off  en=off  dbl_ovrd=off  show_param=off  use_core=on  pipeline=off  use_rpm=on  gen_core=off
      settings: xl_area=[4 8 0 7 0 0 0]
  real : Outport
  imag : Outport  Port=2
  wires:
  ac/1 -> real_sum/1
  bd/1 -> real_sum/2
  bc/1 -> imag_sum/1
  ad/1 -> imag_sum/2
  a/1 -> ad/1, ac/1
  c/1 -> bc/2, ac/2
  b/1 -> bc/1, bd/1
  d/1 -> ad/2, bd/2
  real_sum/1 -> real/1
  imag_sum/1 -> imag/1

== system poco_ref_al_r307/dir_x/ad/vacc_0 ==
  din : Inport  Port=1  LatchInput=off
  new_acc : Inport  Port=2  LatchInput=off
  Adder0 : xbsIndex_r3/AddSub  mode=Addition  precision=User Defined  arith_type="Signed  (2's comp)"  n_bits=32  bin_pt=6  quantization=Truncate  overflow=Wrap  latency=2  explicit_period=on  period=1  use_carryin=off  use_carryout=off  en=off  dbl_ovrd=off  show_param=off  use_core=on  pipeline=off  use_rpm=on  gen_core=off
      settings: xl_area=[0, 0, 0, 0, 0, 0, 0]
  Mux0 : xbsIndex_r3/Mux  inputs=2  precision=Full  arith_type="Signed  (2's comp)"  n_bits=8  bin_pt=2  quantization=Truncate  overflow=Wrap  latency=0  explicit_period=off  period=1  en=off  dbl_ovrd=off  show_param=off  mux_type=off  use_rpm=off  gen_core=off
      settings: xl_area=[0, 0, 0, 0, 0, 0, 0]
  delay_bram : Subsystem  mask(delay_bram){DelayLen=n_chans - 2, bram_latency=2}
      mask prompts: DelayLen "Delay By:"; bram_latency "BRAM Latency"
      mask help: A delay block that uses BRAM for its storage.
      mask init:
      | if (DelayLen <= bram_latency)
      | 	error('delay value must be greater than BRAM Latency');
      | end
      | BitWidth = max(ceil(log2(DelayLen)), 2);
      mask Help: eval('xlWeb([getenv(''MLIB_ROOT''), ''\doc\html\sp_delay_bram\sp_delay_bram.html''])')
  pulse_ext : Subsystem  mask(pulse_ext){pulse_len=n_chans}
      mask prompts: pulse_len "Length of Pulse"
      mask help:
      | Extends a boolean signal to be high for the specified number of clocks after
      | the last high input.
      mask init:
      | bits = ceil(log2(pulse_len+1));
      mask Help: eval('xlWeb([getenv(''MLIB_ROOT''), ''\casper_library\doc\pulse_ext_usage.html''])')
  zero : xbsIndex_r3/Constant  const=0  equ=P=C  arith_type="Signed  (2's comp)"  n_bits=32  bin_pt=6  opselect=C  inp2=PCIN>>17  opr=+  inp1=P  carry=CIN  iostate=0  explicit_period=on  period=1  dbl_ovrd=off
  dout : Outport
  valid : Outport  Port=2
  wires:
  zero/1 -> Mux0/3
  Mux0/1 -> Adder0/2
  pulse_ext/1(out) -> Mux0/1, valid/1
  din/1 -> Adder0/1
  new_acc/1 -> pulse_ext/1(in)
  Adder0/1 -> delay_bram/1(In1)
  delay_bram/1(Out1) -> dout/1, Mux0/2

== system poco_ref_al_r307/dir_x/ad/vacc_1 ==
  din : Inport  Port=1  LatchInput=off
  new_acc : Inport  Port=2  LatchInput=off
  Adder0 : xbsIndex_r3/AddSub  mode=Addition  precision=User Defined  arith_type="Signed  (2's comp)"  n_bits=32  bin_pt=6  quantization=Truncate  overflow=Wrap  latency=2  explicit_period=on  period=1  use_carryin=off  use_carryout=off  en=off  dbl_ovrd=off  show_param=off  use_core=on  pipeline=off  use_rpm=on  gen_core=off
      settings: xl_area=[0, 0, 0, 0, 0, 0, 0]
  Mux0 : xbsIndex_r3/Mux  inputs=2  precision=Full  arith_type="Signed  (2's comp)"  n_bits=8  bin_pt=2  quantization=Truncate  overflow=Wrap  latency=0  explicit_period=off  period=1  en=off  dbl_ovrd=off  show_param=off  mux_type=off  use_rpm=off  gen_core=off
      settings: xl_area=[0, 0, 0, 0, 0, 0, 0]
  delay_bram : Subsystem  mask(delay_bram){DelayLen=n_chans - 2, bram_latency=2}
      mask prompts: DelayLen "Delay By:"; bram_latency "BRAM Latency"
      mask help: A delay block that uses BRAM for its storage.
      mask init:
      | if (DelayLen <= bram_latency)
      | 	error('delay value must be greater than BRAM Latency');
      | end
      | BitWidth = max(ceil(log2(DelayLen)), 2);
      mask Help: eval('xlWeb([getenv(''MLIB_ROOT''), ''\doc\html\sp_delay_bram\sp_delay_bram.html''])')
  pulse_ext : Subsystem  mask(pulse_ext){pulse_len=n_chans}
      mask prompts: pulse_len "Length of Pulse"
      mask help:
      | Extends a boolean signal to be high for the specified number of clocks after
      | the last high input.
      mask init:
      | bits = ceil(log2(pulse_len+1));
      mask Help: eval('xlWeb([getenv(''MLIB_ROOT''), ''\casper_library\doc\pulse_ext_usage.html''])')
  zero : xbsIndex_r3/Constant  const=0  equ=P=C  arith_type="Signed  (2's comp)"  n_bits=32  bin_pt=6  opselect=C  inp2=PCIN>>17  opr=+  inp1=P  carry=CIN  iostate=0  explicit_period=on  period=1  dbl_ovrd=off
  dout : Outport
  valid : Outport  Port=2
  wires:
  delay_bram/1(Out1) -> Mux0/2, dout/1
  Adder0/1 -> delay_bram/1(In1)
  new_acc/1 -> pulse_ext/1(in)
  din/1 -> Adder0/1
  pulse_ext/1(out) -> valid/1, Mux0/1
  Mux0/1 -> Adder0/2
  zero/1 -> Mux0/3
